simulink model "RightCameraAgent"  (Simulink 6.2)
settings: Solver=ode45  StartTime=0.0  StopTime=10.0  RelTol=1e-3
settings Model: LastModifiedBy=suarezjl
settings DataIOCC: SignalLoggingName=sigsOut
settings HardwareCC: TargetUnknown=on

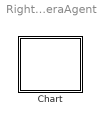
== system RightCameraAgent ==
  Chart : Stateflow chart

== stateflow chart Chart ==
  state Initial
    \\Sally\RightReachDemo\HeadModule\RightCameraAgent\FrameGrabber.Initialize()
    \\Sally\RightReachDemo\HeadModule\RightCameraAgent\FrameGrabber.ObtainImage()
    \\Sally\RightReachDemo\HeadModule\RightCameraAgent\FrameGrabber.ObtainImage()
    \\Sally\RightReachDemo\HeadModule\RightCameraAgent\ColorSegmenter.Initial()
    \\Sally\RightReachDemo\HeadModule\RightCameraAgent\ColorSegmenter.LoadColorModel()
  state Segmentation
    \\Sally\RightReachDemo\HeadModule\RightCameraAgent\FrameGrabber.ObtainImage()
    \\Sally\RightReachDemo\HeadModule\RightCameraAgent\ColorSegmenter.DoSegment()
  (default) -> Initial : Start
  Initial -> Segmentation : Always
  Segmentation -> Segmentation : Always
